simulink model "controllability_test"  (R2021a)
settings: Solver=VariableStepAuto  StartTime=0.0  StopTime=25  RelTol=1e-3
values from neighbouring files (symbols this model uses):
  A = [0 1 0 0 ... (first row only)    [Controllability_of_a_Linear_System.m]    (also in Full_State_Feedback_Control_Design.m = [0 3;2 4]; Implementation_Issues_with_a_FSFB.m = [0 1 0; Introduction_to_Full_State_Feedback_COntrol.m = [0 3;2 4]; Introduction_to_LQR_control.m = [0 1)
  B = [0 ... (first row only)    [Controllability_of_a_Linear_System.m]    (also in Full_State_Feedback_Control_Design.m = [-2 1; 1 1]; Implementation_Issues_with_a_FSFB.m = [0 0; Introduction_to_Full_State_Feedback_COntrol.m = [-2 1; 1 1]; Introduction_to_LQR_control.m)
settings Model: Creator=subhi  LastModifiedBy=subhi

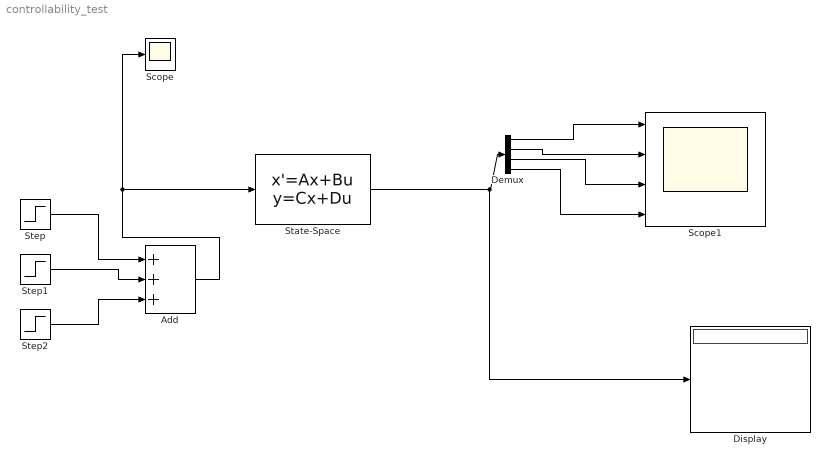
== system controllability_test ==
  Add : Sum  Inputs=+++
  Demux : Demux
  Display : Display
  Scope : Scope
  Scope1 : Scope  NumInputPorts=4
  State-Space : StateSpace  A=A  B=B  C=eye(4)  D=zeros(4,1)  InitialCondition=zeros(4,1)
  Step : Step  Time=5  After=5  SampleTime=1
  Step1 : Step  Time=8  After=-5  SampleTime=0
  Step2 : Step  Time=14  After=5  SampleTime=0
  wires:
  State-Space/1 -> Display/1, Demux/1
  Demux/1 -> Scope1/1
  Demux/4 -> Scope1/4
  Demux/3 -> Scope1/3
  Demux/2 -> Scope1/2
  Step/1 -> Add/1
  Step1/1 -> Add/2
  Step2/1 -> Add/3
  Add/1 -> Scope/1, State-Space/1
